simulink model "EPT"  (R2019b)
settings: Solver=FixedStepDiscrete  StartTime=0.0  StopTime=5  FixedStep=0.005  RelTol=1e-3  EnableMultiTasking=on
PreLoadFcn:
  | try, model_open; catch, disp('Error occurred while executing model pre-load callback: model_open.m'); disp('Please assure that the MATLAB working directory is set to the model directory before opening.'); end
InitFcn:
  | try, model_open; catch, end
undefined symbols (not defined in the file or in its folder): Bridge, GCM, H, ln, raptor_get_param_eval, raptor_get_safe_string, raptor_xcp_function
libraries: Raptor_lib x2810, simulink x374, hdlsllib x19
(part 31 of 45)

== system EPT/Foreground_TimeBase_5ms/CAN/CAN3_exec/PWCU_GENERATOR/PWCU/Cmd_PWCU_Current_PI  ==
  PWCU1_Cout : Inport
  PWCU2_Cout : Inport  Port=2
  PWCU3_Cout : Inport  Port=3
  Ipwcu1_cc_exp : Inport  Port=4
  Ipwcu2_cc_exp : Inport  Port=5
  Ipwcu3_cc_exp : Inport  Port=6
  Enable : EnablePort
  Demux : Demux  Outputs=3
  Gain : Gain  Gain=-1
  Gain2 : Gain  Gain=-1
  Mux : Mux  Inputs=3
  Mux1 : Mux  Inputs=3
  Product : Product
  Product1 : Product
  Saturation Dynamic1 : simulink/Discontinuities/Saturation Dynamic  OutMin=[]  OutMax=[]  OutDataTypeStr=Inherit: Same as second input  OutDataType=fixdt(1, 16)  OutScaling=2^-10  DoSatur=off
  Saturation Dynamic2 : simulink/Discontinuities/Saturation Dynamic  OutMin=[]  OutMax=[]  OutDataTypeStr=Inherit: Same as second input  OutDataType=fixdt(1, 16)  OutScaling=2^-10  DoSatur=off
  Sum : Sum  Inputs=+-
  Sum1 : Sum  Inputs=+++
  Sum2 : Sum  Inputs=+-
  Sum3 : Sum  Inputs=+-
  raptor_adjustment2 : Raptor_lib/Data Storage/raptor_adjustment  paramName='Cal_PWCU_PID_KP'  nameSource=Parameter  initValue=0.5  dataType=double  storage=Calibration  calDispType=Number  calEnum={'False', 'True'}  calGain=1.0  calOffset=0.0  calMax=inf  calMin=-inf  calFormat='-1'  calUnit=''  calHelp=''  calAccess=1  calFunction=raptor_xcp_function(gcb)  calDispHeaders=off  calColHeaders={'Col1' 'Col2' 'Col3'}  calRowHeaders={'Row1' 'Row2' 'Row3'}
      settings: SourceProductName=Raptor
  raptor_adjustment4 : Raptor_lib/Data Storage/raptor_adjustment  paramName='Cal_PWCU_PID_KI'  nameSource=Parameter  initValue=0.4  dataType=double  storage=Calibration  calDispType=Number  calEnum={'False', 'True'}  calGain=1.0  calOffset=0.0  calMax=inf  calMin=-inf  calFormat='-1'  calUnit=''  calHelp=''  calAccess=1  calFunction=raptor_xcp_function(gcb)  calDispHeaders=off  calColHeaders={'Col1' 'Col2' 'Col3'}  calRowHeaders={'Row1' 'Row2' 'Row3'}
      settings: SourceProductName=Raptor
  PWCU1_Cout_Cmd : Outport  VectorParamsAs1DForOutWhenUnconnected=off
  PWCU2_Cout_Cmd : Outport  Port=2  VectorParamsAs1DForOutWhenUnconnected=off
  PWCU3_Cout_Cmd : Outport  Port=3  VectorParamsAs1DForOutWhenUnconnected=off
  wires:
  Sum1/1 -> Demux/1
  Demux/3 -> PWCU3_Cout_Cmd/1
  Demux/1 -> PWCU1_Cout_Cmd/1
  Demux/2 -> PWCU2_Cout_Cmd/1
  Mux/1 -> Product/2, Product1/2
  Sum3/1 -> Mux/3
  Sum2/1 -> Mux/2
  Sum/1 -> Mux/1
  PWCU3_Cout/1 -> Mux1/3, Sum3/2
  Ipwcu3_cc_exp/1 -> Sum3/1
  PWCU2_Cout/1 -> Sum2/2, Mux1/2
  Ipwcu2_cc_exp/1 -> Sum2/1
  raptor_adjustment2/1 -> Gain2/1, Product/1, Saturation Dynamic1/1
  Product1/1 -> Saturation Dynamic2/2
  Ipwcu1_cc_exp/1 -> Sum/1
  PWCU1_Cout/1 -> Sum/2, Mux1/1
  Saturation Dynamic2/1 -> Sum1/2
  Saturation Dynamic1/1 -> Sum1/1
  Product/1 -> Saturation Dynamic1/2
  Gain/1 -> Saturation Dynamic2/3
  Mux1/1 -> Sum1/3
  raptor_adjustment4/1 -> Product1/1, Saturation Dynamic2/1, Gain/1
  Gain2/1 -> Saturation Dynamic1/3

== system EPT/Foreground_TimeBase_5ms/CAN/CAN3_exec/PWCU_GENERATOR/PWCU/CountTrigger1 ==
  Counter : Inport
  Constant1 : Constant  Value=0
  Constant3 : Constant
  CycleTrigger : Subsystem
  Switch : Switch  Threshold=1
  Unit Delay : UnitDelay  SampleTime=-1  HasFrameUpgradeWarning=on
  Tirgger : Outport  VectorParamsAs1DForOutWhenUnconnected=off
  wires:
  Unit Delay/1 -> Switch/2
  CycleTrigger/1(Trigger) -> Unit Delay/1, Tirgger/1
  Counter/1 -> CycleTrigger/2(In2)
  Constant1/1 -> Switch/1
  Constant3/1 -> Switch/3
  Switch/1 -> CycleTrigger/1(In1)

== system EPT/Foreground_TimeBase_5ms/CAN/CAN3_exec/PWCU_GENERATOR/PWCU/Latch1 ==
  Arr_PWCU_Work : Inport
  Arr_PWCU_Temp : Inport  Port=2
  Add : Sum
  Compare To Constant3 : simulink/Logic and Bit Operations/Compare To Constant  relop=>  const=0  OutDataTypeStr=boolean
  Constant3 : Constant
  Divide1 : Product  Inputs=*/
  Min : MinMax  Inputs=2
  NOT : Logic  Operator=NOT  IconShape=distinctive  AllPortsSameDT=off  OutDataTypeStr=boolean
  Product1 : Product
  Product2 : Product
  Product3 : Product
  Subtract3 : Sum  Inputs=+-
  Sum of Elements : Sum  Inputs=+
  Sum of Elements1 : Sum  Inputs=+
  Sum of Elements2 : Sum  Inputs=+
  Switch3 : Switch  Criteria=u2 > Threshold
  raptor_table_1d1 : Raptor_lib/Table Lookup/raptor_table_1d  dataName='PWCUTemp2Ft'  initValue=[0.5,0.75,1,1,1,1,1,1,0.8,0.3,0.10,0,0.0,0]  dataType=double  storage=Calibration  initValueX=[-40,-20,-10,0,10,20,30,50,56,58,60,65,70,80]  dataTypeXY=double  storageXY=Calibration  calVisible=on  showTable=on  calGain=1.0  calOffset=0.0  calMax=Inf  calMin=-Inf  calFormat='-1'  calUnit=''  calHelp=''  showBreakpoint=on  dataNameX=[]  calGainX=1.0  calOffsetX=0.0  calMaxX=Inf  calMinX=-Inf  calFormatX='-1'  calUnitX=''  calHelpX=''  calAccess=1  calFunction=raptor_xcp_function(gcb)  measureEnable=off  mName=[raptor_get_param_eval(gcb,'dataName'), '_Output']
      settings: SourceProductName=Raptor
  PWCUTemp2Ft : Outport
  wires:
  Subtract3/1 -> Product1/2
  Product1/1 -> Sum of Elements/1, Compare To Constant3/1
  Compare To Constant3/1 -> NOT/1, Switch3/2
  Constant3/1 -> Subtract3/1
  Sum of Elements/1 -> Divide1/1
  Arr_PWCU_Work/1 -> Product1/1, Sum of Elements2/1, Product2/1, Product3/2
  Add/1 -> Switch3/3
  Sum of Elements2/1 -> Min/2
  Product3/1 -> PWCUTemp2Ft/1
  Product2/1 -> Switch3/1
  NOT/1 -> Sum of Elements1/1
  Arr_PWCU_Temp/1 -> raptor_table_1d1/1
  raptor_table_1d1/1 -> Subtract3/2, Add/2, Product2/2
  Divide1/1 -> Add/1
  Switch3/1 -> Product3/1
  Sum of Elements1/1 -> Min/1
  Min/1 -> Divide1/2

== system EPT/Foreground_TimeBase_5ms/CAN/CAN3_exec/PWCU_GENERATOR/PWCU/Latch2 ==
  Latch : Inport
  Reset : Inport  Port=2
  Switch1 : Switch  Criteria=u2 > Threshold
  Switch3 : Switch  Criteria=u2 > Threshold
  Unit Delay1 : UnitDelay  SampleTime=-1  HasFrameUpgradeWarning=on
  Output : Outport  VectorParamsAs1DForOutWhenUnconnected=off
  wires:
  Switch1/1 -> Switch3/3
  Latch/1 -> Switch1/2, Switch1/1
  Reset/1 -> Switch3/2
  Switch3/1 -> Unit Delay1/1, Output/1
  Unit Delay1/1 -> Switch1/3

== system EPT/Foreground_TimeBase_5ms/CAN/CAN3_exec/PWCU_GENERATOR/PWCU/PWCU 2_Rx ==
  Trigger : TriggerPort  VariantControl=Variant  PortDimensions=1
  Compare To Constant : simulink/Logic and Bit Operations/Compare To Constant  relop=<=  const=5  OutDataTypeStr=boolean
  Constant : Constant  Value=0.1
  Constant1 : Constant  Value=-40
  Constant2 : Constant
  Convert_Byte2Data : Subsystem
  Convert_Byte2Data1 : Subsystem
  Convert_Byte2Data2 : Subsystem
  Data Type Conversion : DataTypeConversion  OutDataTypeStr=double
  Demux : Demux  Outputs=8
  Demux2 : Demux
  Mux : Mux
  raptor_can_rxraw : Raptor_lib/CAN/raptor_can_rxraw  canBus='CAN3'  extendedId=1  showAge=1  id=hex2dec('180250E5')  idMask=hex2dec('1FFFFFFF')  mailbox=''  queueSize=15
      settings: SourceProductName=Raptor
  raptor_measurement1 : Raptor_lib/Data Storage/raptor_measurement  paramName='Read_PWCU2_Vout'  nameSource=Parameter  calDispType=Number  calEnum={'False', 'True'}  calGain=1.0  calOffset=0.0  calMax=inf  calMin=-inf  calFormat='-1'  calUnit=''  calHelp=''  calAccess=1  calFunction=raptor_xcp_function(gcb)  calVisible=on
      settings: SourceProductName=Raptor
  raptor_measurement2 : Raptor_lib/Data Storage/raptor_measurement  paramName='Read_PWCU2_Cout'  nameSource=Parameter  calDispType=Number  calEnum={'False', 'True'}  calGain=1.0  calOffset=0.0  calMax=inf  calMin=-inf  calFormat='-1'  calUnit=''  calHelp=''  calAccess=1  calFunction=raptor_xcp_function(gcb)  calVisible=on
      settings: SourceProductName=Raptor
  raptor_measurement3 : Raptor_lib/Data Storage/raptor_measurement  paramName='Read_PWCU2_Status'  nameSource=Parameter  calDispType=Number  calEnum={'False', 'True'}  calGain=1.0  calOffset=0.0  calMax=inf  calMin=-inf  calFormat='-1'  calUnit=''  calHelp=''  calAccess=1  calFunction=raptor_xcp_function(gcb)  calVisible=on
      settings: SourceProductName=Raptor
  raptor_measurement9 : Raptor_lib/Data Storage/raptor_measurement  paramName='PWCU2_Age'  nameSource=Parameter  calDispType=Number  calEnum={'False', 'True'}  calGain=1.0  calOffset=0.0  calMax=inf  calMin=-inf  calFormat='-1'  calUnit=''  calHelp=''  calAccess=1  calFunction=raptor_xcp_function(gcb)  calVisible=on
      settings: SourceProductName=Raptor
  "PWCU2_Cout " : Outport  VectorParamsAs1DForOutWhenUnconnected=off
  "PWCU2_Temp " : Outport  Port=2  VectorParamsAs1DForOutWhenUnconnected=off
  PWCU2_Work : Outport  Port=3  VectorParamsAs1DForOutWhenUnconnected=off
  wires:
  Demux2/2 -> "PWCU2_Cout "/1, raptor_measurement2/1
  Demux2/1 -> raptor_measurement1/1
  Mux/1 -> Demux2/1
  Demux2/3 -> raptor_measurement3/1
  Data Type Conversion/1 -> Mux/3
  Demux/5 -> Data Type Conversion/1
  Convert_Byte2Data2/1(Data) -> Mux/4
  Convert_Byte2Data1/1(Data) -> Mux/2
  Convert_Byte2Data/1(Data) -> Mux/1
  Demux/1 -> Convert_Byte2Data/1(HighByte)
  raptor_can_rxraw/5 -> Demux/1
  Constant/1 -> Convert_Byte2Data1/4(Factor), Convert_Byte2Data/4(Factor)
  Constant1/1 -> Convert_Byte2Data2/3(Offset)
  Demux/2 -> Convert_Byte2Data/2(LowByte)
  Demux/3 -> Convert_Byte2Data1/1(HighByte)
  Demux/4 -> Convert_Byte2Data1/2(LowByte)
  Constant2/1 -> Convert_Byte2Data2/4(Factor)
  Demux/6 -> Convert_Byte2Data2/2(LowByte)
  raptor_can_rxraw/1 -> Compare To Constant/1, raptor_measurement9/1
  Compare To Constant/1 -> PWCU2_Work/1
  Demux2/4 -> "PWCU2_Temp "/1

== system EPT/Foreground_TimeBase_5ms/CAN/CAN3_exec/PWCU_GENERATOR/PWCU/PWCU 3_Rx ==
  Trigger : TriggerPort  VariantControl=Variant  PortDimensions=1
  Compare To Constant : simulink/Logic and Bit Operations/Compare To Constant  relop=<=  const=5  OutDataTypeStr=boolean
  Constant : Constant  Value=0.1
  Constant1 : Constant  Value=-40
  Constant2 : Constant
  Convert_Byte2Data : Subsystem
  Convert_Byte2Data1 : Subsystem
  Convert_Byte2Data2 : Subsystem
  Data Type Conversion : DataTypeConversion  OutDataTypeStr=double
  Demux : Demux  Outputs=8
  Demux2 : Demux
  Mux : Mux
  raptor_can_rxraw : Raptor_lib/CAN/raptor_can_rxraw  canBus='CAN3'  extendedId=1  showAge=1  id=hex2dec('180350E5')  idMask=hex2dec('1FFFFFFF')  mailbox=''  queueSize=15
      settings: SourceProductName=Raptor
  raptor_measurement1 : Raptor_lib/Data Storage/raptor_measurement  paramName='Read_PWCU3_Vout'  nameSource=Parameter  calDispType=Number  calEnum={'False', 'True'}  calGain=1.0  calOffset=0.0  calMax=inf  calMin=-inf  calFormat='-1'  calUnit=''  calHelp=''  calAccess=1  calFunction=raptor_xcp_function(gcb)  calVisible=on
      settings: SourceProductName=Raptor
  raptor_measurement2 : Raptor_lib/Data Storage/raptor_measurement  paramName='Read_PWCU3_Cout'  nameSource=Parameter  calDispType=Number  calEnum={'False', 'True'}  calGain=1.0  calOffset=0.0  calMax=inf  calMin=-inf  calFormat='-1'  calUnit=''  calHelp=''  calAccess=1  calFunction=raptor_xcp_function(gcb)  calVisible=on
      settings: SourceProductName=Raptor
  raptor_measurement3 : Raptor_lib/Data Storage/raptor_measurement  paramName='Read_PWCU3_Status'  nameSource=Parameter  calDispType=Number  calEnum={'False', 'True'}  calGain=1.0  calOffset=0.0  calMax=inf  calMin=-inf  calFormat='-1'  calUnit=''  calHelp=''  calAccess=1  calFunction=raptor_xcp_function(gcb)  calVisible=on
      settings: SourceProductName=Raptor
  raptor_measurement9 : Raptor_lib/Data Storage/raptor_measurement  paramName='PWCU3_Age'  nameSource=Parameter  calDispType=Number  calEnum={'False', 'True'}  calGain=1.0  calOffset=0.0  calMax=inf  calMin=-inf  calFormat='-1'  calUnit=''  calHelp=''  calAccess=1  calFunction=raptor_xcp_function(gcb)  calVisible=on
      settings: SourceProductName=Raptor
  "PWCU3_Cout " : Outport  VectorParamsAs1DForOutWhenUnconnected=off
  "PWCU3_Temp " : Outport  Port=2  VectorParamsAs1DForOutWhenUnconnected=off
  PWCU3_Work : Outport  Port=3  VectorParamsAs1DForOutWhenUnconnected=off
  wires:
  Demux/6 -> Convert_Byte2Data2/2(LowByte)
  Constant2/1 -> Convert_Byte2Data2/4(Factor)
  Demux/4 -> Convert_Byte2Data1/2(LowByte)
  Demux/3 -> Convert_Byte2Data1/1(HighByte)
  Demux/2 -> Convert_Byte2Data/2(LowByte)
  Constant1/1 -> Convert_Byte2Data2/3(Offset)
  Constant/1 -> Convert_Byte2Data/4(Factor), Convert_Byte2Data1/4(Factor)
  raptor_can_rxraw/5 -> Demux/1
  Demux/1 -> Convert_Byte2Data/1(HighByte)
  Convert_Byte2Data/1(Data) -> Mux/1
  Convert_Byte2Data1/1(Data) -> Mux/2
  Convert_Byte2Data2/1(Data) -> Mux/4
  Demux/5 -> Data Type Conversion/1
  Data Type Conversion/1 -> Mux/3
  Demux2/3 -> raptor_measurement3/1
  Mux/1 -> Demux2/1
  Demux2/1 -> raptor_measurement1/1
  Demux2/2 -> raptor_measurement2/1, "PWCU3_Cout "/1
  Compare To Constant/1 -> PWCU3_Work/1
  raptor_can_rxraw/1 -> Compare To Constant/1, raptor_measurement9/1
  Demux2/4 -> "PWCU3_Temp "/1

== system EPT/Foreground_TimeBase_5ms/CAN/CAN3_exec/PWCU_GENERATOR/PWCU/PWCU1_Rx ==
  Trigger : TriggerPort  VariantControl=Variant  PortDimensions=1
  Compare To Constant : simulink/Logic and Bit Operations/Compare To Constant  relop=<=  const=5  OutDataTypeStr=boolean
  Constant : Constant  Value=0.1
  Constant1 : Constant  Value=-40
  Constant2 : Constant
  Convert_Byte2Data : Subsystem
  Convert_Byte2Data1 : Subsystem
  Convert_Byte2Data2 : Subsystem
  Data Type Conversion : DataTypeConversion  OutDataTypeStr=double
  Demux : Demux  Outputs=8
  Demux2 : Demux
  Mux : Mux
  raptor_can_rxraw : Raptor_lib/CAN/raptor_can_rxraw  canBus='CAN3'  extendedId=1  showAge=1  id=hex2dec('180150E5')  idMask=hex2dec('1FFFFFFF')  mailbox=''  queueSize=15
      settings: SourceProductName=Raptor
  raptor_measurement1 : Raptor_lib/Data Storage/raptor_measurement  paramName='Read_PWCU1_Vout'  nameSource=Parameter  calDispType=Number  calEnum={'False', 'True'}  calGain=1.0  calOffset=0.0  calMax=inf  calMin=-inf  calFormat='-1'  calUnit=''  calHelp=''  calAccess=1  calFunction=raptor_xcp_function(gcb)  calVisible=on
      settings: SourceProductName=Raptor
  raptor_measurement2 : Raptor_lib/Data Storage/raptor_measurement  paramName='Read_PWCU1_Cout'  nameSource=Parameter  calDispType=Number  calEnum={'False', 'True'}  calGain=1.0  calOffset=0.0  calMax=inf  calMin=-inf  calFormat='-1'  calUnit=''  calHelp=''  calAccess=1  calFunction=raptor_xcp_function(gcb)  calVisible=on
      settings: SourceProductName=Raptor
  raptor_measurement3 : Raptor_lib/Data Storage/raptor_measurement  paramName='Read_PWCU1_Status'  nameSource=Parameter  calDispType=Number  calEnum={'False', 'True'}  calGain=1.0  calOffset=0.0  calMax=inf  calMin=-inf  calFormat='-1'  calUnit=''  calHelp=''  calAccess=1  calFunction=raptor_xcp_function(gcb)  calVisible=on
      settings: SourceProductName=Raptor
  raptor_measurement9 : Raptor_lib/Data Storage/raptor_measurement  paramName='PWCU1_Age'  nameSource=Parameter  calDispType=Number  calEnum={'False', 'True'}  calGain=1.0  calOffset=0.0  calMax=inf  calMin=-inf  calFormat='-1'  calUnit=''  calHelp=''  calAccess=1  calFunction=raptor_xcp_function(gcb)  calVisible=on
      settings: SourceProductName=Raptor
  "PWCU1_Cout " : Outport  VectorParamsAs1DForOutWhenUnconnected=off
  "PWCU1_Temp " : Outport  Port=2  VectorParamsAs1DForOutWhenUnconnected=off
  PWCU1_Work : Outport  Port=3  VectorParamsAs1DForOutWhenUnconnected=off
  wires:
  Constant2/1 -> Convert_Byte2Data2/4(Factor)
  Demux/6 -> Convert_Byte2Data2/2(LowByte)
  Demux/4 -> Convert_Byte2Data1/2(LowByte)
  Demux/3 -> Convert_Byte2Data1/1(HighByte)
  Demux/2 -> Convert_Byte2Data/2(LowByte)
  Constant1/1 -> Convert_Byte2Data2/3(Offset)
  Constant/1 -> Convert_Byte2Data1/4(Factor), Convert_Byte2Data/4(Factor)
  raptor_can_rxraw/5 -> Demux/1
  Demux/1 -> Convert_Byte2Data/1(HighByte)
  Convert_Byte2Data/1(Data) -> Mux/1
  Convert_Byte2Data1/1(Data) -> Mux/2
  Convert_Byte2Data2/1(Data) -> Mux/4
  Demux/5 -> Data Type Conversion/1
  Data Type Conversion/1 -> Mux/3
  Demux2/3 -> raptor_measurement3/1
  Mux/1 -> Demux2/1
  Demux2/1 -> raptor_measurement1/1
  Demux2/2 -> "PWCU1_Cout "/1, raptor_measurement2/1
  raptor_can_rxraw/1 -> Compare To Constant/1, raptor_measurement9/1
  Compare To Constant/1 -> PWCU1_Work/1
  Demux2/4 -> "PWCU1_Temp "/1

== system EPT/Foreground_TimeBase_5ms/CAN/CAN3_exec/PWCU_GENERATOR/PWCU/PWCU1_Tx ==
  PWCU1_Icmd : Inport
  PI_On : Inport  Port=2
  PWCU1_EN : Inport  Port=3
  Trigger : TriggerPort  VariantControl=Variant  PortDimensions=1
  Constant4 : Constant  OutDataTypeStr=boolean
  Constant6 : Constant  Value=8  OutDataTypeStr=uint8
  Constant7 : Constant  Value=0.1
  Convert_Data2Byte : Subsystem
  Convert_Data2Byte1 : Subsystem
  Data Type Conversion{1..6} (6 alike) : DataTypeConversion  OutDataTypeStr=uint8
  Mux1 : Mux  Inputs=8
  Switch : Switch  Criteria=u2 > Threshold
  raptor_adjustment2 : Raptor_lib/Data Storage/raptor_adjustment  paramName='Cal_PWCU1_TxID'  nameSource=Parameter  initValue=hex2dec('1801E5F4')  dataType=uint32  storage=Calibration  calDispType=Number  calEnum={'False', 'True'}  calGain=1.0  calOffset=0.0  calMax=inf  calMin=-inf  calFormat='-1'  calUnit=''  calHelp=''  calAccess=1  calFunction=raptor_xcp_function(gcb)  calDispHeaders=off  calColHeaders={'Col1' 'Col2' 'Col3'}  calRowHeaders={'Row1' 'Row2' 'Row3'}
      settings: SourceProductName=Raptor
  raptor_adjustment3 : Raptor_lib/Data Storage/raptor_adjustment  paramName='PWCU1_Cmd_CHGV'  nameSource=Parameter  initValue=110  dataType=double  storage=Calibration  calDispType=Number  calEnum={'False', 'True'}  calGain=1.0  calOffset=0.0  calMax=inf  calMin=-inf  calFormat='-1'  calUnit=''  calHelp=''  calAccess=1  calFunction=raptor_xcp_function(gcb)  calDispHeaders=off  calColHeaders={'Col1' 'Col2' 'Col3'}  calRowHeaders={'Row1' 'Row2' 'Row3'}
      settings: SourceProductName=Raptor
  raptor_adjustment4 : Raptor_lib/Data Storage/raptor_adjustment  paramName='PWCU1_Cmd_CHGA'  nameSource=Parameter  initValue=0.00  dataType=double  storage=Calibration  calDispType=Number  calEnum={'False', 'True'}  calGain=1.0  calOffset=0.0  calMax=inf  calMin=-inf  calFormat='-1'  calUnit=''  calHelp=''  calAccess=1  calFunction=raptor_xcp_function(gcb)  calDispHeaders=off  calColHeaders={'Col1' 'Col2' 'Col3'}  calRowHeaders={'Row1' 'Row2' 'Row3'}
      settings: SourceProductName=Raptor
  raptor_adjustment6 : Raptor_lib/Data Storage/raptor_adjustment  paramName='PWCU1_Status'  nameSource=Parameter  initValue=0.00  dataType=double  storage=Calibration  calDispType=Number  calEnum={'False', 'True'}  calGain=1.0  calOffset=0.0  calMax=inf  calMin=-inf  calFormat='-1'  calUnit=''  calHelp=''  calAccess=1  calFunction=raptor_xcp_function(gcb)  calDispHeaders=off  calColHeaders={'Col1' 'Col2' 'Col3'}  calRowHeaders={'Row1' 'Row2' 'Row3'}
      settings: SourceProductName=Raptor
  raptor_can_txraw2 : Raptor_lib/CAN/raptor_can_txraw  canBus='CAN3'  queueSize=1  showIdTypePort=1  idTypeSelectValues=Standard|Extended  idTypeSelect=Standard
      settings: SourceProductName=Raptor
  wires:
  Convert_Data2Byte/2(LowByte) -> Data Type Conversion1/1
  Convert_Data2Byte1/1(HighByte) -> Data Type Conversion2/1
  Constant6/1 -> raptor_can_txraw2/3
  Data Type Conversion5/1 -> Mux1/6
  Mux1/1 -> raptor_can_txraw2/4
  raptor_adjustment2/1 -> raptor_can_txraw2/2
  Constant7/1 -> Convert_Data2Byte1/2(Factor), Convert_Data2Byte/2(Factor)
  Data Type Conversion2/1 -> Mux1/3
  Data Type Conversion4/1 -> Mux1/5
  Convert_Data2Byte1/2(LowByte) -> Data Type Conversion3/1
  Data Type Conversion1/1 -> Mux1/2
  raptor_adjustment3/1 -> Convert_Data2Byte/1(Data)
  raptor_adjustment6/1 -> Data Type Conversion5/1
  Data Type Conversion3/1 -> Mux1/4
  Constant4/1 -> raptor_can_txraw2/1
  Data Type Conversion6/1 -> Mux1/1
  Convert_Data2Byte/1(HighByte) -> Data Type Conversion6/1
  raptor_adjustment4/1 -> Switch/3
  Switch/1 -> Convert_Data2Byte1/1(Data)
  PWCU1_Icmd/1 -> Switch/1
  PI_On/1 -> Switch/2
  PWCU1_EN/1 -> Data Type Conversion4/1

== system EPT/Foreground_TimeBase_5ms/CAN/CAN3_exec/PWCU_GENERATOR/PWCU/PWCU2_Tx ==
  PWCU2_Icmd : Inport
  PI_On : Inport  Port=2
  PWCU2_EN : Inport  Port=3
  Trigger : TriggerPort  VariantControl=Variant  PortDimensions=1
  Constant3 : Constant  OutDataTypeStr=boolean
  Constant5 : Constant  Value=8  OutDataTypeStr=uint8
  Constant8 : Constant  Value=0.1
  Convert_Data2Byte : Subsystem
  Convert_Data2Byte1 : Subsystem
  Data Type Conversion{1..5,14} (6 alike) : DataTypeConversion  OutDataTypeStr=uint8
  Mux2 : Mux  Inputs=8
  Switch : Switch  Criteria=u2 > Threshold
  raptor_adjustment1 : Raptor_lib/Data Storage/raptor_adjustment  paramName='PWCU2_Cmd_CHGV'  nameSource=Parameter  initValue=110  dataType=double  storage=Calibration  calDispType=Number  calEnum={'False', 'True'}  calGain=1.0  calOffset=0.0  calMax=inf  calMin=-inf  calFormat='-1'  calUnit=''  calHelp=''  calAccess=1  calFunction=raptor_xcp_function(gcb)  calDispHeaders=off  calColHeaders={'Col1' 'Col2' 'Col3'}  calRowHeaders={'Row1' 'Row2' 'Row3'}
      settings: SourceProductName=Raptor
  raptor_adjustment10 : Raptor_lib/Data Storage/raptor_adjustment  paramName='PWCU2_Status'  nameSource=Parameter  initValue=0.00  dataType=double  storage=Calibration  calDispType=Number  calEnum={'False', 'True'}  calGain=1.0  calOffset=0.0  calMax=inf  calMin=-inf  calFormat='-1'  calUnit=''  calHelp=''  calAccess=1  calFunction=raptor_xcp_function(gcb)  calDispHeaders=off  calColHeaders={'Col1' 'Col2' 'Col3'}  calRowHeaders={'Row1' 'Row2' 'Row3'}
      settings: SourceProductName=Raptor
  raptor_adjustment7 : Raptor_lib/Data Storage/raptor_adjustment  paramName='Cal_PWCU2_TxID'  nameSource=Parameter  initValue=hex2dec('1802E5F4')  dataType=uint32  storage=Calibration  calDispType=Number  calEnum={'False', 'True'}  calGain=1.0  calOffset=0.0  calMax=inf  calMin=-inf  calFormat='-1'  calUnit=''  calHelp=''  calAccess=1  calFunction=raptor_xcp_function(gcb)  calDispHeaders=off  calColHeaders={'Col1' 'Col2' 'Col3'}  calRowHeaders={'Row1' 'Row2' 'Row3'}
      settings: SourceProductName=Raptor
  raptor_adjustment8 : Raptor_lib/Data Storage/raptor_adjustment  paramName='PWCU2_Cmd_CHGA'  nameSource=Parameter  initValue=0.00  dataType=double  storage=Calibration  calDispType=Number  calEnum={'False', 'True'}  calGain=1.0  calOffset=0.0  calMax=inf  calMin=-inf  calFormat='-1'  calUnit=''  calHelp=''  calAccess=1  calFunction=raptor_xcp_function(gcb)  calDispHeaders=off  calColHeaders={'Col1' 'Col2' 'Col3'}  calRowHeaders={'Row1' 'Row2' 'Row3'}
      settings: SourceProductName=Raptor
  raptor_can_txraw1 : Raptor_lib/CAN/raptor_can_txraw  canBus='CAN3'  queueSize=1  showIdTypePort=1  idTypeSelectValues=Standard|Extended  idTypeSelect=Standard
      settings: SourceProductName=Raptor
  wires:
  Data Type Conversion14/1 -> Mux2/1
  Data Type Conversion1/1 -> Mux2/2
  Mux2/1 -> raptor_can_txraw1/4
  Constant8/1 -> Convert_Data2Byte1/2(Factor), Convert_Data2Byte/2(Factor)
  raptor_adjustment1/1 -> Convert_Data2Byte/1(Data)
  Data Type Conversion3/1 -> Mux2/4
  Constant5/1 -> raptor_can_txraw1/3
  Constant3/1 -> raptor_can_txraw1/1
  Data Type Conversion5/1 -> Mux2/6
  PWCU2_EN/1 -> Data Type Conversion4/1
  Convert_Data2Byte1/2(LowByte) -> Data Type Conversion3/1
  Data Type Conversion2/1 -> Mux2/3
  Data Type Conversion4/1 -> Mux2/5
  raptor_adjustment10/1 -> Data Type Conversion5/1
  Convert_Data2Byte/2(LowByte) -> Data Type Conversion1/1
  Convert_Data2Byte1/1(HighByte) -> Data Type Conversion2/1
  raptor_adjustment7/1 -> raptor_can_txraw1/2
  Convert_Data2Byte/1(HighByte) -> Data Type Conversion14/1
  raptor_adjustment8/1 -> Switch/3
  Switch/1 -> Convert_Data2Byte1/1(Data)
  PWCU2_Icmd/1 -> Switch/1
  PI_On/1 -> Switch/2

== system EPT/Foreground_TimeBase_5ms/CAN/CAN3_exec/PWCU_GENERATOR/PWCU/PWCU3_Tx3 ==
  PWCU3_Icmd : Inport
  PI_On : Inport  Port=2
  PWCU3_EN : Inport  Port=3
  Trigger : TriggerPort  VariantControl=Variant  PortDimensions=1
  Constant3 : Constant  OutDataTypeStr=boolean
  Constant5 : Constant  Value=8  OutDataTypeStr=uint8
  Constant8 : Constant  Value=0.1
  Convert_Data2Byte : Subsystem
  Convert_Data2Byte1 : Subsystem
  Data Type Conversion{1..5,14} (6 alike) : DataTypeConversion  OutDataTypeStr=uint8
  Mux2 : Mux  Inputs=8
  Switch : Switch  Criteria=u2 > Threshold
  raptor_adjustment1 : Raptor_lib/Data Storage/raptor_adjustment  paramName='PWCU3_Cmd_CHGV'  nameSource=Parameter  initValue=110  dataType=double  storage=Calibration  calDispType=Number  calEnum={'False', 'True'}  calGain=1.0  calOffset=0.0  calMax=inf  calMin=-inf  calFormat='-1'  calUnit=''  calHelp=''  calAccess=1  calFunction=raptor_xcp_function(gcb)  calDispHeaders=off  calColHeaders={'Col1' 'Col2' 'Col3'}  calRowHeaders={'Row1' 'Row2' 'Row3'}
      settings: SourceProductName=Raptor
  raptor_adjustment10 : Raptor_lib/Data Storage/raptor_adjustment  paramName='PWCU3_Status'  nameSource=Parameter  initValue=0.00  dataType=double  storage=Calibration  calDispType=Number  calEnum={'False', 'True'}  calGain=1.0  calOffset=0.0  calMax=inf  calMin=-inf  calFormat='-1'  calUnit=''  calHelp=''  calAccess=1  calFunction=raptor_xcp_function(gcb)  calDispHeaders=off  calColHeaders={'Col1' 'Col2' 'Col3'}  calRowHeaders={'Row1' 'Row2' 'Row3'}
      settings: SourceProductName=Raptor
  raptor_adjustment7 : Raptor_lib/Data Storage/raptor_adjustment  paramName='Cal_PWCU3_TxID'  nameSource=Parameter  initValue=hex2dec('1803E5F4')  dataType=uint32  storage=Calibration  calDispType=Number  calEnum={'False', 'True'}  calGain=1.0  calOffset=0.0  calMax=inf  calMin=-inf  calFormat='-1'  calUnit=''  calHelp=''  calAccess=1  calFunction=raptor_xcp_function(gcb)  calDispHeaders=off  calColHeaders={'Col1' 'Col2' 'Col3'}  calRowHeaders={'Row1' 'Row2' 'Row3'}
      settings: SourceProductName=Raptor
  raptor_adjustment8 : Raptor_lib/Data Storage/raptor_adjustment  paramName='PWCU3_Cmd_CHGA'  nameSource=Parameter  initValue=0.00  dataType=double  storage=Calibration  calDispType=Number  calEnum={'False', 'True'}  calGain=1.0  calOffset=0.0  calMax=inf  calMin=-inf  calFormat='-1'  calUnit=''  calHelp=''  calAccess=1  calFunction=raptor_xcp_function(gcb)  calDispHeaders=off  calColHeaders={'Col1' 'Col2' 'Col3'}  calRowHeaders={'Row1' 'Row2' 'Row3'}
      settings: SourceProductName=Raptor
  raptor_can_txraw1 : Raptor_lib/CAN/raptor_can_txraw  canBus='CAN3'  queueSize=1  showIdTypePort=1  idTypeSelectValues=Standard|Extended  idTypeSelect=Standard
      settings: SourceProductName=Raptor
  wires:
  PI_On/1 -> Switch/2
  PWCU3_Icmd/1 -> Switch/1
  Switch/1 -> Convert_Data2Byte1/1(Data)
  raptor_adjustment8/1 -> Switch/3
  Convert_Data2Byte/1(HighByte) -> Data Type Conversion14/1
  raptor_adjustment7/1 -> raptor_can_txraw1/2
  Convert_Data2Byte1/1(HighByte) -> Data Type Conversion2/1
  Convert_Data2Byte/2(LowByte) -> Data Type Conversion1/1
  raptor_adjustment10/1 -> Data Type Conversion5/1
  Data Type Conversion4/1 -> Mux2/5
  Data Type Conversion2/1 -> Mux2/3
  Convert_Data2Byte1/2(LowByte) -> Data Type Conversion3/1
  PWCU3_EN/1 -> Data Type Conversion4/1
  Data Type Conversion5/1 -> Mux2/6
  Constant3/1 -> raptor_can_txraw1/1
  Constant5/1 -> raptor_can_txraw1/3
  Data Type Conversion3/1 -> Mux2/4
  raptor_adjustment1/1 -> Convert_Data2Byte/1(Data)
  Constant8/1 -> Convert_Data2Byte/2(Factor), Convert_Data2Byte1/2(Factor)
  Mux2/1 -> raptor_can_txraw1/4
  Data Type Conversion1/1 -> Mux2/2
  Data Type Conversion14/1 -> Mux2/1

== system EPT/Foreground_TimeBase_5ms/CAN/CAN3_exec/PWCU_GENERATOR/PWCU/Subsystem ==
  note: Applictation
  "Cmd_PWCU_Current_PI " : Subsystem
  Constant13 : Constant  Value=0
  CountTrigger2 : Subsystem
  Demux : Demux  Outputs=3
  Divide : Product  Inputs=*/
  Divide1 : Product  Inputs=*/
  Divide2 : Product  Inputs=***
  Gain : Gain  Gain=1000
  Latch3 : Subsystem
  Latch4 : Subsystem
  Latch5 : Subsystem
  Mux : Mux  Inputs=3
  Relational Operator10 : RelationalOperator  Operator=<  OutDataTypeStr=boolean  RndMeth=Simplest
  Relational Operator5 : RelationalOperator  Operator=>  OutDataTypeStr=boolean  RndMeth=Simplest
  Relational Operator6 : RelationalOperator  Operator=<  OutDataTypeStr=boolean  RndMeth=Simplest
  Relational Operator7 : RelationalOperator  Operator=>  OutDataTypeStr=boolean  RndMeth=Simplest
  Relational Operator8 : RelationalOperator  Operator=<  OutDataTypeStr=boolean  RndMeth=Simplest
  Relational Operator9 : RelationalOperator  Operator=>  OutDataTypeStr=boolean  RndMeth=Simplest
  Saturation : Saturate  UpperLimit=30  LowerLimit=0
  Sum : Sum  Inputs=+++
  Switch : Switch  Criteria=u2 > Threshold
  Switch2 : Switch  Criteria=u2 > Threshold
  Switch3 : Switch  Criteria=u2 > Threshold
  raptor_adjustment1 : Raptor_lib/Data Storage/raptor_adjustment  paramName='Cal_GeneratorPW_LowCondition'  nameSource=Parameter  initValue=3  dataType=double  storage=Calibration  calDispType=Number  calEnum={'False', 'True'}  calGain=1.0  calOffset=0.0  calMax=inf  calMin=-inf  calFormat='-1'  calUnit=''  calHelp=''  calAccess=1  calFunction=raptor_xcp_function(gcb)  calDispHeaders=off  calColHeaders={'Col1' 'Col2' 'Col3'}  calRowHeaders={'Row1' 'Row2' 'Row3'}
      settings: SourceProductName=Raptor
  raptor_adjustment10 : Raptor_lib/Data Storage/raptor_adjustment  paramName='Cal_GeneratorPW_Low_SoC_Region1'  nameSource=Parameter  initValue=40  dataType=double  storage=Calibration  calDispType=Number  calEnum={'False', 'True'}  calGain=1.0  calOffset=0.0  calMax=inf  calMin=-inf  calFormat='-1'  calUnit=''  calHelp=''  calAccess=1  calFunction=raptor_xcp_function(gcb)  calDispHeaders=off  calColHeaders={'Col1' 'Col2' 'Col3'}  calRowHeaders={'Row1' 'Row2' 'Row3'}
      settings: SourceProductName=Raptor
  raptor_adjustment11 : Raptor_lib/Data Storage/raptor_adjustment  paramName='Cal_GeneratorPW_Low_SoC_Region2'  nameSource=Parameter  initValue=45  dataType=double  storage=Calibration  calDispType=Number  calEnum={'False', 'True'}  calGain=1.0  calOffset=0.0  calMax=inf  calMin=-inf  calFormat='-1'  calUnit=''  calHelp=''  calAccess=1  calFunction=raptor_xcp_function(gcb)  calDispHeaders=off  calColHeaders={'Col1' 'Col2' 'Col3'}  calRowHeaders={'Row1' 'Row2' 'Row3'}
      settings: SourceProductName=Raptor
  raptor_adjustment2 : Raptor_lib/Data Storage/raptor_adjustment  paramName='Cal_GeneratorPW_MidCondition'  nameSource=Parameter  initValue=5  dataType=double  storage=Calibration  calDispType=Number  calEnum={'False', 'True'}  calGain=1.0  calOffset=0.0  calMax=inf  calMin=-inf  calFormat='-1'  calUnit=''  calHelp=''  calAccess=1  calFunction=raptor_xcp_function(gcb)  calDispHeaders=off  calColHeaders={'Col1' 'Col2' 'Col3'}  calRowHeaders={'Row1' 'Row2' 'Row3'}
      settings: SourceProductName=Raptor
  raptor_adjustment3 : Raptor_lib/Data Storage/raptor_adjustment  paramName='PWCU_PI_Time'  nameSource=Parameter  initValue=30  dataType=double  storage=Calibration  calDispType=Number  calEnum={'False', 'True'}  calGain=1.0  calOffset=0.0  calMax=inf  calMin=-inf  calFormat='-1'  calUnit=''  calHelp=''  calAccess=1  calFunction=raptor_xcp_function(gcb)  calDispHeaders=off  calColHeaders={'Col1' 'Col2' 'Col3'}  calRowHeaders={'Row1' 'Row2' 'Row3'}
      settings: SourceProductName=Raptor
  raptor_adjustment5 : Raptor_lib/Data Storage/raptor_adjustment  paramName='Cal_GeneratorPW_HighCondition'  nameSource=Parameter  initValue=8  dataType=double  storage=Calibration  calDispType=Number  calEnum={'False', 'True'}  calGain=1.0  calOffset=0.0  calMax=inf  calMin=-inf  calFormat='-1'  calUnit=''  calHelp=''  calAccess=1  calFunction=raptor_xcp_function(gcb)  calDispHeaders=off  calColHeaders={'Col1' 'Col2' 'Col3'}  calRowHeaders={'Row1' 'Row2' 'Row3'}
      settings: SourceProductName=Raptor
  raptor_adjustment6 : Raptor_lib/Data Storage/raptor_adjustment  paramName='Cal_GeneratorPW_High_SoC_Region1'  nameSource=Parameter  initValue=80  dataType=double  storage=Calibration  calDispType=Number  calEnum={'False', 'True'}  calGain=1.0  calOffset=0.0  calMax=inf  calMin=-inf  calFormat='-1'  calUnit=''  calHelp=''  calAccess=1  calFunction=raptor_xcp_function(gcb)  calDispHeaders=off  calColHeaders={'Col1' 'Col2' 'Col3'}  calRowHeaders={'Row1' 'Row2' 'Row3'}
      settings: SourceProductName=Raptor
  raptor_adjustment7 : Raptor_lib/Data Storage/raptor_adjustment  paramName='Cal_GeneratorPW_High_SoC_Region2'  nameSource=Parameter  initValue=85  dataType=double  storage=Calibration  calDispType=Number  calEnum={'False', 'True'}  calGain=1.0  calOffset=0.0  calMax=inf  calMin=-inf  calFormat='-1'  calUnit=''  calHelp=''  calAccess=1  calFunction=raptor_xcp_function(gcb)  calDispHeaders=off  calColHeaders={'Col1' 'Col2' 'Col3'}  calRowHeaders={'Row1' 'Row2' 'Row3'}
      settings: SourceProductName=Raptor
  raptor_adjustment8 : Raptor_lib/Data Storage/raptor_adjustment  paramName='Cal_GeneratorPW_SOC_Region'  nameSource=Parameter  initValue=70  dataType=double  storage=Calibration  calDispType=Number  calEnum={'False', 'True'}  calGain=1.0  calOffset=0.0  calMax=inf  calMin=-inf  calFormat='-1'  calUnit=''  calHelp=''  calAccess=1  calFunction=raptor_xcp_function(gcb)  calDispHeaders=off  calColHeaders={'Col1' 'Col2' 'Col3'}  calRowHeaders={'Row1' 'Row2' 'Row3'}
      settings: SourceProductName=Raptor
  raptor_adjustment9 : Raptor_lib/Data Storage/raptor_adjustment  paramName='Cal_GeneratorPW_Mid_SoC_Region2'  nameSource=Parameter  initValue=75  dataType=double  storage=Calibration  calDispType=Number  calEnum={'False', 'True'}  calGain=1.0  calOffset=0.0  calMax=inf  calMin=-inf  calFormat='-1'  calUnit=''  calHelp=''  calAccess=1  calFunction=raptor_xcp_function(gcb)  calDispHeaders=off  calColHeaders={'Col1' 'Col2' 'Col3'}  calRowHeaders={'Row1' 'Row2' 'Row3'}
      settings: SourceProductName=Raptor
  raptor_data_read1 : Raptor_lib/Data Storage/raptor_data_read  dataName='EPT_BPOBU_SOC'  dataShape=Scalar  idxSource=Input  idxRow=1  idxCol=1
      settings: SourceProductName=Raptor
  raptor_data_read10 : Raptor_lib/Data Storage/raptor_data_read  dataName='Ft_CHG_Vcell'  dataShape=Scalar  idxSource=Input  idxRow=1  idxCol=1
      settings: SourceProductName=Raptor
  raptor_data_read2 : Raptor_lib/Data Storage/raptor_data_read  dataName='EPT_HV_BUS_VOLT'  dataShape=Scalar  idxSource=Input  idxRow=1  idxCol=1
      settings: SourceProductName=Raptor
  raptor_measurement1 : Raptor_lib/Data Storage/raptor_measurement  paramName='Ipwcu3_cc_exp'  nameSource=Parameter  calDispType=Number  calEnum={'False', 'True'}  calGain=1.0  calOffset=0.0  calMax=inf  calMin=-inf  calFormat='-1'  calUnit=''  calHelp=''  calAccess=1  calFunction=raptor_xcp_function(gcb)  calVisible=on
      settings: SourceProductName=Raptor
  raptor_measurement2 : Raptor_lib/Data Storage/raptor_measurement  paramName='Ipwcu2_cc_exp'  nameSource=Parameter  calDispType=Number  calEnum={'False', 'True'}  calGain=1.0  calOffset=0.0  calMax=inf  calMin=-inf  calFormat='-1'  calUnit=''  calHelp=''  calAccess=1  calFunction=raptor_xcp_function(gcb)  calVisible=on
      settings: SourceProductName=Raptor
  raptor_measurement9 : Raptor_lib/Data Storage/raptor_measurement  paramName='Ipwcu1_cc_exp'  nameSource=Parameter  calDispType=Number  calEnum={'False', 'True'}  calGain=1.0  calOffset=0.0  calMax=inf  calMin=-inf  calFormat='-1'  calUnit=''  calHelp=''  calAccess=1  calFunction=raptor_xcp_function(gcb)  calVisible=on
      settings: SourceProductName=Raptor
  raptor_override : Raptor_lib/Data Storage/raptor_override  paramName='Cal_PWCU_EPT_BPOBU_SOC'  nameSource=Parameter  measurement=None  calDispType=Number  calEnum={'False', 'True'}  calGain=1.0  calOffset=0.0  calMax=inf  calMin=-inf  calFormat='-1'  calUnit=''  calHelp=''  calAccess=1  calFunction=[raptor_xcp_function(gcb) '|' raptor_get_param_eval(gcb, 'paramName') '_Override']
      settings: SourceProductName=Raptor
  raptor_override1 : Raptor_lib/Data Storage/raptor_override  paramName='Cal_PWCU1_Temp'  nameSource=Parameter  measurement=None  calDispType=Number  calEnum={'False', 'True'}  calGain=1.0  calOffset=0.0  calMax=inf  calMin=-inf  calFormat='-1'  calUnit=''  calHelp=''  calAccess=1  calFunction=[raptor_xcp_function(gcb) '|' raptor_get_param_eval(gcb, 'paramName') '_Override']
      settings: SourceProductName=Raptor
  raptor_override2 : Raptor_lib/Data Storage/raptor_override  paramName='Cal_PWCU2_Temp'  nameSource=Parameter  measurement=None  calDispType=Number  calEnum={'False', 'True'}  calGain=1.0  calOffset=0.0  calMax=inf  calMin=-inf  calFormat='-1'  calUnit=''  calHelp=''  calAccess=1  calFunction=[raptor_xcp_function(gcb) '|' raptor_get_param_eval(gcb, 'paramName') '_Override']
      settings: SourceProductName=Raptor
  raptor_override3 : Raptor_lib/Data Storage/raptor_override  paramName='Cal_PWCU3_Temp'  nameSource=Parameter  measurement=None  calDispType=Number  calEnum={'False', 'True'}  calGain=1.0  calOffset=0.0  calMax=inf  calMin=-inf  calFormat='-1'  calUnit=''  calHelp=''  calAccess=1  calFunction=[raptor_xcp_function(gcb) '|' raptor_get_param_eval(gcb, 'paramName') '_Override']
      settings: SourceProductName=Raptor
  raptor_table_1d3 : Raptor_lib/Table Lookup/raptor_table_1d  dataName='PWCUTemp2Ft'  initValue=[0.5,0.75,1,1,1,1,1,1,0.8,0.3,0.10,0,0.0,0]  dataType=double  storage=Calibration  initValueX=[-40,-20,-10,0,10,20,30,50,56,58,60,65,70,80]  dataTypeXY=double  storageXY=Calibration  calVisible=on  showTable=on  calGain=1.0  calOffset=0.0  calMax=Inf  calMin=-Inf  calFormat='-1'  calUnit=''  calHelp=''  showBreakpoint=on  dataNameX=[]  calGainX=1.0  calOffsetX=0.0  calMaxX=Inf  calMinX=-Inf  calFormatX='-1'  calUnitX=''  calHelpX=''  calAccess=1  calFunction=raptor_xcp_function(gcb)  measureEnable=off  mName=[raptor_get_param_eval(gcb,'dataName'), '_Output']
      settings: SourceProductName=Raptor
  wires:
  Divide/1 -> Divide1/1
  Demux/3 -> raptor_measurement1/1, [Ipwcu3_cc_exp]
  [PWCU1_Temp] -> raptor_override1/1
  Relational Operator10/1 -> Latch5/1(Latch)
  Relational Operator8/1 -> Latch4/1(Latch)
  raptor_adjustment7/1 -> Relational Operator9/2
  Demux/2 -> raptor_measurement2/1, [Ipwcu2_cc_exp]
  [Ipwcu2_cc_exp] -> "Cmd_PWCU_Current_PI "/5(Ipwcu2_cc_exp)
  [PWCU2_Temp] -> raptor_override2/1
  raptor_adjustment3/1 -> CountTrigger2/1(Counter)
  raptor_adjustment9/1 -> Relational Operator5/2
  raptor_data_read10/1 -> Divide2/3
  [PWCU3_Temp] -> raptor_override3/1
  [Ipwcu3_cc_exp] -> "Cmd_PWCU_Current_PI "/6(Ipwcu3_cc_exp)
  "Cmd_PWCU_Current_PI "/2(PWCU2_Cout_Cmd) -> [PWCU2_Icmd]
  raptor_adjustment11/1 -> Relational Operator7/2
  Saturation/1 -> Demux/1
  [PWCU3_Cout] -> "Cmd_PWCU_Current_PI "/3(PWCU3_Cout)
  [PWCU2_Work] -> Sum/2
  Gain/1 -> Divide/1
  raptor_adjustment8/1 -> Relational Operator6/2
  Switch3/1 -> Switch/3
  raptor_override/1 -> Relational Operator7/1, Relational Operator10/1, Relational Operator9/1, Relational Operator6/1, Relational Operator5/1, Relational Operator8/1
  [Ipwcu1_cc_exp] -> "Cmd_PWCU_Current_PI "/4(Ipwcu1_cc_exp)
  Switch/1 -> Switch2/3
  raptor_adjustment6/1 -> Relational Operator10/2
  raptor_override3/1 -> Mux/3
  Switch2/1 -> Gain/1
  Latch3/1(Output) -> Switch/2
  raptor_data_read2/1 -> Divide/2
  [PWCU1_Cout] -> "Cmd_PWCU_Current_PI "/1(PWCU1_Cout)
  Divide1/1 -> Divide2/1
  Relational Operator9/1 -> Latch5/2(Reset)
  "Cmd_PWCU_Current_PI "/3(PWCU3_Cout_Cmd) -> [PWCU3_Icmd]
  Latch5/1(Output) -> Switch3/2
  "Cmd_PWCU_Current_PI "/1(PWCU1_Cout_Cmd) -> [PWCU1_Icmd]
  Relational Operator7/1 -> Latch4/2(Reset)
  Mux/1 -> raptor_table_1d3/1
  raptor_override2/1 -> Mux/2
  raptor_adjustment10/1 -> Relational Operator8/2
  raptor_adjustment5/1 -> Switch2/1
  Demux/1 -> [Ipwcu1_cc_exp], raptor_measurement9/1
  CountTrigger2/1(Tirgger) -> "Cmd_PWCU_Current_PI "/Enable
  [PWCU2_Cout] -> "Cmd_PWCU_Current_PI "/2(PWCU2_Cout)
  Divide2/1 -> Saturation/1
  [PWCU1_Work] -> Sum/1
  raptor_adjustment2/1 -> Switch/1
  [PWCU3_Work] -> Sum/3
  raptor_data_read1/1 -> raptor_override/1
  Relational Operator5/1 -> Latch3/2(Reset)
  Latch4/1(Output) -> Switch2/2
  Constant13/1 -> Switch3/3
  Relational Operator6/1 -> Latch3/1(Latch)
  Sum/1 -> Divide1/2
  raptor_adjustment1/1 -> Switch3/1
  raptor_table_1d3/1 -> Divide2/2
  raptor_override1/1 -> Mux/1

== system EPT/Foreground_TimeBase_5ms/CAN/CAN3_exec/SEVCON_MCU /CountTrigger1/CycleTrigger ==
  In1 : Inport
  In2 : Inport  Port=2
  Add : Sum
  Add1 : Sum
  Add2 : Sum  Inputs=+-
  Constant1 : Constant
  Constant2 : Constant  Value=0
  Constant3 : Constant
  Data Type Conversion1 : DataTypeConversion
  Data Type Conversion2 : DataTypeConversion
  Display : Display
  Relational Operator1 : RelationalOperator  OutDataTypeStr=boolean  RndMeth=Simplest
  Scope : Scope
  Scope1 : Scope
  Scope2 : Scope
  Switch : Switch  Threshold=1
  Unit Delay : UnitDelay  SampleTime=-1  HasFrameUpgradeWarning=on
  Unit Delay1 : UnitDelay  SampleTime=-1  HasFrameUpgradeWarning=on
  Trigger : Outport  VectorParamsAs1DForOutWhenUnconnected=off
  wires:
  Constant3/1 -> Add2/2
  In2/1 -> Add2/1
  Add2/1 -> Data Type Conversion1/1
  Data Type Conversion2/1 -> Switch/2, Add/2
  Constant2/1 -> Switch/3
  Data Type Conversion1/1 -> Relational Operator1/2
  Relational Operator1/1 -> Trigger/1, Scope2/1
  Constant1/1 -> Add1/2
  Unit Delay1/1 -> Add1/1
  Add1/1 -> Display/1, Unit Delay1/1, Scope/1
  Switch/1 -> Unit Delay/1, Scope1/1, Relational Operator1/1
  Unit Delay/1 -> Add/1
  In1/1 -> Data Type Conversion2/1
  Add/1 -> Switch/1

== system EPT/Foreground_TimeBase_5ms/CAN/CAN3_exec/SEVCON_MCU /CountTrigger2/CycleTrigger ==
  In1 : Inport
  In2 : Inport  Port=2
  Add : Sum
  Add1 : Sum
  Add2 : Sum  Inputs=+-
  Constant1 : Constant
  Constant2 : Constant  Value=0
  Constant3 : Constant
  Data Type Conversion1 : DataTypeConversion
  Data Type Conversion2 : DataTypeConversion
  Display : Display
  Relational Operator1 : RelationalOperator  OutDataTypeStr=boolean  RndMeth=Simplest
  Scope : Scope
  Scope1 : Scope
  Scope2 : Scope
  Switch : Switch  Threshold=1
  Unit Delay : UnitDelay  SampleTime=-1  HasFrameUpgradeWarning=on
  Unit Delay1 : UnitDelay  SampleTime=-1  HasFrameUpgradeWarning=on
  Trigger : Outport  VectorParamsAs1DForOutWhenUnconnected=off
  wires:
  Constant3/1 -> Add2/2
  In2/1 -> Add2/1
  Add2/1 -> Data Type Conversion1/1
  Data Type Conversion2/1 -> Switch/2, Add/2
  Constant2/1 -> Switch/3
  Data Type Conversion1/1 -> Relational Operator1/2
  Relational Operator1/1 -> Trigger/1, Scope2/1
  Constant1/1 -> Add1/2
  Unit Delay1/1 -> Add1/1
  Add1/1 -> Display/1, Unit Delay1/1, Scope/1
  Switch/1 -> Unit Delay/1, Scope1/1, Relational Operator1/1
  Unit Delay/1 -> Add/1
  In1/1 -> Data Type Conversion2/1
  Add/1 -> Switch/1

== system EPT/Foreground_TimeBase_5ms/CAN/CAN3_exec/SEVCON_MCU /SEVCON_Error_Code/Convert_Byte2Data1 ==
  LowByte : Inport
  HighByte : Inport  Port=2
  Factor : Inport  Port=3
  Offset : Inport  Port=4
  Add1 : Sum
  Add2 : Sum
  Constant10 : Constant  Value=256
  Data Type Conversion10 : DataTypeConversion  OutDataTypeStr=int16
  Divide1 : Product  Inputs=**
  Divide6 : Product  Inputs=**
  Data(int16) : Outport  VectorParamsAs1DForOutWhenUnconnected=off
  wires:
  Factor/1 -> Divide1/2
  Data Type Conversion10/1 -> Data(int16)/1
  Add2/1 -> Divide1/1
  Divide1/1 -> Add1/1
  Constant10/1 -> Divide6/2
  HighByte/1 -> Divide6/1
  Add1/1 -> Data Type Conversion10/1
  LowByte/1 -> Add2/1
  Divide6/1 -> Add2/2
  Offset/1 -> Add1/2

== system EPT/Foreground_TimeBase_5ms/CAN/CAN3_exec/SEVCON_MCU /SEVCON_Error_Code/Convert_Byte2Data2 ==
  LowByte : Inport
  HighByte : Inport  Port=2
  Factor : Inport  Port=3
  Offset : Inport  Port=4
  Add1 : Sum
  Add2 : Sum
  Constant10 : Constant  Value=256
  Data Type Conversion10 : DataTypeConversion  OutDataTypeStr=int16
  Divide1 : Product  Inputs=**
  Divide6 : Product  Inputs=**
  Data(int16) : Outport  VectorParamsAs1DForOutWhenUnconnected=off
  wires:
  Offset/1 -> Add1/2
  Divide6/1 -> Add2/2
  LowByte/1 -> Add2/1
  Add1/1 -> Data Type Conversion10/1
  HighByte/1 -> Divide6/1
  Constant10/1 -> Divide6/2
  Divide1/1 -> Add1/1
  Add2/1 -> Divide1/1
  Data Type Conversion10/1 -> Data(int16)/1
  Factor/1 -> Divide1/2

== system EPT/Foreground_TimeBase_5ms/CAN/CAN3_exec/SEVCON_MCU /SEVCON_Error_Code/EPT_MCU_FAULT_LEVEL ==
  Bitwise AND : simulink/Logic and Bit Operations/Bitwise Operator  logicop=AND  UseBitMask=on  BitMask=hex2dec('FF00')  BitMaskRealWorld=Stored Integer
  Constant : Constant  Value=hex2dec('4400')
  Constant1 : Constant  Value=hex2dec('4700')
  Constant10 : Constant
  Constant11 : Constant  Value=2
  Constant12 : Constant  Value=3
  Constant13 : Constant  Value=4
  Constant14 : Constant  Value=5
  Constant15 : Constant  Value=0
  Constant2 : Constant  Value=hex2dec('4800')
  Constant3 : Constant  Value=hex2dec('4B00')
  Constant4 : Constant  Value=hex2dec('4C00')
  Constant5 : Constant  Value=hex2dec('4F00')
  Constant6 : Constant  Value=hex2dec('5000')
  Constant7 : Constant  Value=hex2dec('5300')
  Constant8 : Constant  Value=hex2dec('5400')
  Constant9 : Constant  Value=hex2dec('5700')
  Logical Operator{,1..4} (5 alike) : Logic  AllPortsSameDT=off  OutDataTypeStr=boolean
  Relational Operator{,2,4,6,8} (5 alike) : RelationalOperator  OutDataTypeStr=boolean  RndMeth=Simplest
  Relational Operator{1,3,5,7,9} (5 alike) : RelationalOperator  Operator=<=  OutDataTypeStr=boolean  RndMeth=Simplest
  Switch{,1..4} (5 alike) : Switch  Criteria=u2 > Threshold
  raptor_data_def3 : Raptor_lib/Data Storage/raptor_data_def  dataName='EPT_MCU_FAULT_LEVEL'  initValue=0  dataType=double  storage=Volatile (RAM)  calVisible=on  calType=Measurement  calDispType=Number  calEnum={'False', 'True'}  calGain=1.0  calOffset=0  calMin=-inf  calMax=inf  calFormat='-1'  calUnit=''  calHelp=''  calAccess=1  calFunction=raptor_xcp_function(gcb)  calDispHeaders=off  calColHeaders={'Col1' 'Col2' 'Col3'}  calRowHeaders={'Row1' 'Row2' 'Row3'}
      settings: SourceProductName=Raptor
  raptor_data_read : Raptor_lib/Data Storage/raptor_data_read  dataName='EPT_MCU_FAULT_ID'  dataShape=Scalar  idxSource=Input  idxRow=1  idxCol=1
      settings: SourceProductName=Raptor
  raptor_data_write2 : Raptor_lib/Data Storage/raptor_data_write  dataName='EPT_MCU_FAULT_LEVEL'  dataShape=Scalar  idxSource=Input Port  idxRow=1  idxCol=1
      settings: SourceProductName=Raptor
  wires:
  raptor_data_read/1 -> Bitwise AND/1
  Relational Operator/1 -> Logical Operator/1
  Relational Operator1/1 -> Logical Operator/2
  Constant/1 -> Relational Operator/2
  Constant1/1 -> Relational Operator1/2
  Constant3/1 -> Relational Operator3/2
  Constant2/1 -> Relational Operator2/2
  Relational Operator3/1 -> Logical Operator1/2
  Relational Operator2/1 -> Logical Operator1/1
  Relational Operator4/1 -> Logical Operator2/1
  Relational Operator5/1 -> Logical Operator2/2
  Constant4/1 -> Relational Operator4/2
  Constant5/1 -> Relational Operator5/2
  Constant7/1 -> Relational Operator7/2
  Constant6/1 -> Relational Operator6/2
  Relational Operator7/1 -> Logical Operator3/2
  Relational Operator6/1 -> Logical Operator3/1
  Bitwise AND/1 -> Relational Operator1/1, Relational Operator2/1, Relational Operator4/1, Relational Operator8/1, Relational Operator9/1, Relational Operator7/1, Relational Operator6/1, Relational Operator5/1, Relational Operator3/1, Relational Operator/1
  Relational Operator8/1 -> Logical Operator4/1
  Relational Operator9/1 -> Logical Operator4/2
  Constant8/1 -> Relational Operator8/2
  Constant9/1 -> Relational Operator9/2
  Logical Operator/1 -> Switch/2
  Logical Operator1/1 -> Switch1/2
  Logical Operator3/1 -> Switch3/2
  Logical Operator4/1 -> Switch4/2
  Switch/1 -> Switch1/3
  Switch1/1 -> Switch2/3
  Switch2/1 -> Switch3/3
  Switch3/1 -> Switch4/3
  Constant10/1 -> Switch/1
  Constant11/1 -> Switch1/1
  Logical Operator2/1 -> Switch2/2
  Constant12/1 -> Switch2/1
  Constant13/1 -> Switch3/1
  Constant14/1 -> Switch4/1
  Constant15/1 -> Switch/3
  Switch4/1 -> raptor_data_write2/1
